simulink model "chap04_CA2"  (R2021a)
settings: Solver=FixedStepDiscrete  StartTime=0.0  StopTime=30  FixedStep=0.001  RelTol=1e-3
undefined symbols (not defined in the file): DiscIntNeverNeededParam
libraries: simulink x4
(part 3 of 3)

== system chap04_CA2/Subsystem/Subsystem5/Subsystem6 ==
  xx3 : Inport
  xx1 : Inport  Port=2
  xx4 : Inport  Port=3
  xx5 : Inport  Port=4
  vx3 : Inport  Port=5
  vx1 : Inport  Port=6
  vx4 : Inport  Port=7
  vx5 : Inport  Port=8
  Add : Sum
  Add{1,4,6,8} (4 alike) : Sum  Inputs=-+
  Add2 : Sum  Inputs=+-
  Add5 : Sum  Inputs=+++
  Add7 : Sum  Inputs=+-
  Add9 : Sum  Inputs=+++
  Constant{,1,3,6} (4 alike) : Constant  Value=1.0
  Constant2 : Constant  Value=7/9
  Constant4 : Constant  Value=0.5
  Constant5 : Constant  Value=1.5
  Constant7 : Constant  Value=0.5
  Constant8 : Constant  Value=1.5
  Constant9 : Constant  Value=3
  Divide : Product  Inputs=*/
  Gain : Gain  Gain=-1
  Math Function1 : Math  Operator=pow  SignedPower=on  SaturateOnIntegerOverflow=on
  Product{1,3..9} (8 alike) : Product
  p3x : Outport
  wires:
  Product8/1 -> Add9/2
  Product9/1 -> Add9/3
  Constant6/1 -> Product8/1
  Add8/1 -> Product8/2
  vx3/1 -> Add6/2, Add8/2, Add7/1
  Constant7/1 -> Product9/2
  Add7/1 -> Product9/1
  vx4/1 -> Add8/1
  vx1/1 -> Add7/2
  vx5/1 -> Add6/1
  Constant8/1 -> Product7/1
  Add6/1 -> Product7/2
  Product7/1 -> Add9/1
  Product3/1 -> Add5/1
  Add1/1 -> Product3/2
  Constant5/1 -> Product3/1
  xx5/1 -> Add1/1
  xx1/1 -> Add2/2
  xx4/1 -> Add4/1
  Add5/1 -> Product6/2
  Add2/1 -> Product5/1
  Product1/1 -> Add/2
  Constant1/1 -> Product1/1
  Constant/1 -> Product6/1
  Product6/1 -> Add/1
  Constant4/1 -> Product5/2
  xx3/1 -> Add2/1, Add4/2, Add1/2
  Add4/1 -> Product4/2
  Constant3/1 -> Product4/1
  Product5/1 -> Add5/3
  Product4/1 -> Add5/2
  Add9/1 -> Product1/2
  Math Function1/1 -> Gain/1
  Constant9/1 -> Divide/2
  Divide/1 -> Math Function1/1
  Add/1 -> Divide/1
  Constant2/1 -> Math Function1/2
  Gain/1 -> p3x/1

== system chap04_CA2/Subsystem/Subsystem5/Subsystem7 ==
  vy3 : Inport
  uty : Inport  Port=2
  gain : Inport  Port=3
  Add1 : Sum  Inputs=--+
  Constant : Constant  Value=0.08
  Constant2 : Constant  Value=15
  Product : Product
  Product1 : Product
  Product2 : Product
  Subsystem : Subsystem
  Subtract : Sum  Inputs=+-
  Tanh : Trigonometry  Operator=tanh
  ux : Outport
  wires:
  Subtract/1 -> Product2/1, Product1/2
  Constant/1 -> Product1/1
  Product1/1 -> Add1/1
  Constant2/1 -> Product2/2
  [A] -> Add1/3
  gain/1 -> Product/2
  Tanh/1 -> Product/1
  Product2/1 -> Tanh/1
  vy3/1 -> Subtract/1
  Product/1 -> Add1/2
  Subsystem/1(Out1) -> Subtract/2
  uty/1 -> Subsystem/1(zt3), [A]
  Add1/1 -> ux/1

== system chap04_CA2/Subsystem/Subsystem5/Subsystem8 ==
  vz3 : Inport
  utz : Inport  Port=2
  gain : Inport  Port=3
  Add1 : Sum  Inputs=--+
  Constant : Constant  Value=0.08
  Constant2 : Constant  Value=15
  Product : Product
  Product1 : Product
  Product2 : Product
  Subsystem : Subsystem
  Subtract : Sum  Inputs=+-
  Tanh : Trigonometry  Operator=tanh
  ux : Outport
  wires:
  Add1/1 -> ux/1
  utz/1 -> [A], Subsystem/1(zt3)
  Subsystem/1(Out1) -> Subtract/2
  Product/1 -> Add1/2
  vz3/1 -> Subtract/1
  Product2/1 -> Tanh/1
  Tanh/1 -> Product/1
  gain/1 -> Product/2
  [A] -> Add1/3
  Constant2/1 -> Product2/2
  Product1/1 -> Add1/1
  Constant/1 -> Product1/1
  Subtract/1 -> Product1/2, Product2/1

== system chap04_CA2/Subsystem2/Subsystem7/Subsystem1 ==
  Abs1 : Abs
  Add : Sum  Inputs=+++
  Constant : Constant  Value=0.8
  Constant1 : Constant  Value=0.1
  Constant3 : Constant  Value=0.1
  Delay1 : Delay
  Delay2 : Delay  DelayLength=1
  Product{1..4} (4 alike) : Product
  Random Number1 : RandomNumber  Mean=0.75  Variance=0.5  Seed=2  SampleTime=0.01
  Repeating Sequence Interpolated2 : simulink/Sources/Repeating Sequence Interpolated  OutValues=[0.5 0.25 0.4 0.35 0.1].'  TimeValues=[0 0.1 0.5 0.6 1].'  LookUpMeth=Use Input Nearest  tsamp=1  OutMin=[]  OutMax=[]  OutDataTypeStr=double  OutputDataTypeScalingMode=double  OutDataType=fixdt(0,8)  OutScaling=2^-10
  Scope : Scope
  Out2 : Outport
  wires:
  Delay1/1 -> Product2/1
  Delay2/1 -> Product1/1
  Constant/1 -> Product2/2
  Constant3/1 -> Product1/2
  Constant1/1 -> Product3/2
  Product3/1 -> Add/1
  Product1/1 -> Add/2
  Product2/1 -> Add/3
  Product4/1 -> Product3/1
  Add/1 -> Out2/1, Delay1/1, Delay2/1
  Abs1/1 -> Product4/1, Scope/1
  Random Number1/1 -> Abs1/1
  Repeating Sequence Interpolated2/1 -> Product4/2

== system chap04_CA2/Subsystem2/Subsystem7/Subsystem2 ==
  In2 : Inport
  Add : Sum  Inputs=+++
  Constant : Constant  Value=0.8
  Constant1 : Constant  Value=0.1
  Constant3 : Constant  Value=0.1
  Delay1 : Delay
  Delay2 : Delay  DelayLength=1
  Product1 : Product
  Product2 : Product
  Product3 : Product
  Out2 : Outport
  wires:
  Add/1 -> Delay2/1, Delay1/1, Out2/1
  In2/1 -> Product3/1
  Product2/1 -> Add/3
  Product1/1 -> Add/2
  Product3/1 -> Add/1
  Constant1/1 -> Product3/2
  Constant3/1 -> Product1/2
  Constant/1 -> Product2/2
  Delay2/1 -> Product1/1
  Delay1/1 -> Product2/1

== system chap04_CA2/Subsystem2/Subsystem7/Subsystem3 ==
  In2 : Inport
  Add : Sum  Inputs=+++
  Constant : Constant  Value=0.8
  Constant1 : Constant  Value=0.1
  Constant3 : Constant  Value=0.1
  Delay1 : Delay
  Delay2 : Delay  DelayLength=1
  Product1 : Product
  Product2 : Product
  Product3 : Product
  Out2 : Outport
  wires:
  Delay1/1 -> Product2/1
  Delay2/1 -> Product1/1
  Constant/1 -> Product2/2
  Constant3/1 -> Product1/2
  Constant1/1 -> Product3/2
  Product3/1 -> Add/1
  Product1/1 -> Add/2
  Product2/1 -> Add/3
  In2/1 -> Product3/1
  Add/1 -> Out2/1, Delay1/1, Delay2/1

== system chap04_CA2/Subsystem2/Subsystem7/Subsystem4 ==
  In2 : Inport
  Add : Sum  Inputs=+++
  Constant : Constant  Value=0.8
  Constant1 : Constant  Value=0.1
  Constant3 : Constant  Value=0.1
  Delay1 : Delay
  Delay2 : Delay  DelayLength=1
  Product1 : Product
  Product2 : Product
  Product3 : Product
  Out2 : Outport
  wires:
  Add/1 -> Delay2/1, Delay1/1, Out2/1
  In2/1 -> Product3/1
  Product2/1 -> Add/3
  Product1/1 -> Add/2
  Product3/1 -> Add/1
  Constant1/1 -> Product3/2
  Constant3/1 -> Product1/2
  Constant/1 -> Product2/2
  Delay2/1 -> Product1/1
  Delay1/1 -> Product2/1

== system chap04_CA2/Subsystem/Subsystem/Subsystem4/Subsystem ==
  zt3 : Inport
  Constant4 : Constant  Value=0
  Discrete-Time Integrator : DiscreteIntegrator  SampleTime=-1  UpperSaturationLimit=100  LowerSaturationLimit=-100  ICPrevOutput=DiscIntNeverNeededParam  ICPrevScaledInput=DiscIntNeverNeededParam
  Logical Operator : Logic  AllPortsSameDT=off  OutDataTypeStr=boolean
  MATLAB Function : MATLAB Function  TreatAsAtomicUnit=on
  Relational Operator : RelationalOperator  Operator===  OutDataTypeStr=boolean  RndMeth=Simplest
  Saturation : Saturate  UpperLimit=5  LowerLimit=-5
  Sign : Signum
  Sign1 : Signum
  Switch : Switch  Criteria=u2 > Threshold
  Out1 : Outport
  wires:
  MATLAB Function/1(y) -> Logical Operator/1
  Relational Operator/1 -> Logical Operator/2
  Constant4/1 -> Switch/1
  Sign1/1 -> Relational Operator/1
  zt3/1 -> Sign1/1, Switch/3
  Saturation/1 -> Out1/1, MATLAB Function/2(u2)
  Discrete-Time Integrator/1 -> Saturation/1, MATLAB Function/1(u1), Sign/1
  Sign/1 -> Relational Operator/2
  Logical Operator/1 -> Switch/2
  Switch/1 -> Discrete-Time Integrator/1

== system chap04_CA2/Subsystem/Subsystem/Subsystem7/Subsystem ==
  zt3 : Inport
  Constant4 : Constant  Value=0
  Discrete-Time Integrator : DiscreteIntegrator  SampleTime=-1  UpperSaturationLimit=100  LowerSaturationLimit=-100  ICPrevOutput=DiscIntNeverNeededParam  ICPrevScaledInput=DiscIntNeverNeededParam
  Logical Operator : Logic  AllPortsSameDT=off  OutDataTypeStr=boolean
  MATLAB Function : MATLAB Function  TreatAsAtomicUnit=on
  Relational Operator : RelationalOperator  Operator===  OutDataTypeStr=boolean  RndMeth=Simplest
  Saturation : Saturate  UpperLimit=5  LowerLimit=-5
  Sign : Signum
  Sign1 : Signum
  Switch : Switch  Criteria=u2 > Threshold
  Out1 : Outport
  wires:
  Switch/1 -> Discrete-Time Integrator/1
  Logical Operator/1 -> Switch/2
  Sign/1 -> Relational Operator/2
  Discrete-Time Integrator/1 -> Sign/1, MATLAB Function/1(u1), Saturation/1
  Saturation/1 -> MATLAB Function/2(u2), Out1/1
  zt3/1 -> Switch/3, Sign1/1
  Sign1/1 -> Relational Operator/1
  Constant4/1 -> Switch/1
  Relational Operator/1 -> Logical Operator/2
  MATLAB Function/1(y) -> Logical Operator/1

== system chap04_CA2/Subsystem/Subsystem/Subsystem8/Subsystem ==
  zt3 : Inport
  Constant4 : Constant  Value=0
  Discrete-Time Integrator : DiscreteIntegrator  SampleTime=-1  UpperSaturationLimit=100  LowerSaturationLimit=-100  ICPrevOutput=DiscIntNeverNeededParam  ICPrevScaledInput=DiscIntNeverNeededParam
  Logical Operator : Logic  AllPortsSameDT=off  OutDataTypeStr=boolean
  MATLAB Function : MATLAB Function  TreatAsAtomicUnit=on
  Relational Operator : RelationalOperator  Operator===  OutDataTypeStr=boolean  RndMeth=Simplest
  Saturation : Saturate  UpperLimit=5  LowerLimit=-5
  Sign : Signum
  Sign1 : Signum
  Switch : Switch  Criteria=u2 > Threshold
  Out1 : Outport
  wires:
  MATLAB Function/1(y) -> Logical Operator/1
  Relational Operator/1 -> Logical Operator/2
  Constant4/1 -> Switch/1
  Sign1/1 -> Relational Operator/1
  zt3/1 -> Sign1/1, Switch/3
  Saturation/1 -> Out1/1, MATLAB Function/2(u2)
  Discrete-Time Integrator/1 -> Saturation/1, MATLAB Function/1(u1), Sign/1
  Sign/1 -> Relational Operator/2
  Logical Operator/1 -> Switch/2
  Switch/1 -> Discrete-Time Integrator/1

== system chap04_CA2/Subsystem/Subsystem1/Subsystem4/Subsystem ==
  zt3 : Inport
  Constant4 : Constant  Value=0
  Discrete-Time Integrator : DiscreteIntegrator  SampleTime=-1  UpperSaturationLimit=100  LowerSaturationLimit=-100  ICPrevOutput=DiscIntNeverNeededParam  ICPrevScaledInput=DiscIntNeverNeededParam
  Logical Operator : Logic  AllPortsSameDT=off  OutDataTypeStr=boolean
  MATLAB Function : MATLAB Function  TreatAsAtomicUnit=on
  Relational Operator : RelationalOperator  Operator===  OutDataTypeStr=boolean  RndMeth=Simplest
  Saturation : Saturate  UpperLimit=5  LowerLimit=-5
  Sign : Signum
  Sign1 : Signum
  Switch : Switch  Criteria=u2 > Threshold
  Out1 : Outport
  wires:
  MATLAB Function/1(y) -> Logical Operator/1
  Relational Operator/1 -> Logical Operator/2
  Constant4/1 -> Switch/1
  Sign1/1 -> Relational Operator/1
  zt3/1 -> Sign1/1, Switch/3
  Saturation/1 -> Out1/1, MATLAB Function/2(u2)
  Discrete-Time Integrator/1 -> Saturation/1, MATLAB Function/1(u1), Sign/1
  Sign/1 -> Relational Operator/2
  Logical Operator/1 -> Switch/2
  Switch/1 -> Discrete-Time Integrator/1

== system chap04_CA2/Subsystem/Subsystem1/Subsystem7/Subsystem ==
  zt3 : Inport
  Constant4 : Constant  Value=0
  Discrete-Time Integrator : DiscreteIntegrator  SampleTime=-1  UpperSaturationLimit=100  LowerSaturationLimit=-100  ICPrevOutput=DiscIntNeverNeededParam  ICPrevScaledInput=DiscIntNeverNeededParam
  Logical Operator : Logic  AllPortsSameDT=off  OutDataTypeStr=boolean
  MATLAB Function : MATLAB Function  TreatAsAtomicUnit=on
  Relational Operator : RelationalOperator  Operator===  OutDataTypeStr=boolean  RndMeth=Simplest
  Saturation : Saturate  UpperLimit=5  LowerLimit=-5
  Sign : Signum
  Sign1 : Signum
  Switch : Switch  Criteria=u2 > Threshold
  Out1 : Outport
  wires:
  Switch/1 -> Discrete-Time Integrator/1
  Logical Operator/1 -> Switch/2
  Sign/1 -> Relational Operator/2
  Discrete-Time Integrator/1 -> Sign/1, MATLAB Function/1(u1), Saturation/1
  Saturation/1 -> MATLAB Function/2(u2), Out1/1
  zt3/1 -> Switch/3, Sign1/1
  Sign1/1 -> Relational Operator/1
  Constant4/1 -> Switch/1
  Relational Operator/1 -> Logical Operator/2
  MATLAB Function/1(y) -> Logical Operator/1

== system chap04_CA2/Subsystem/Subsystem1/Subsystem8/Subsystem ==
  zt3 : Inport
  Constant4 : Constant  Value=0
  Discrete-Time Integrator : DiscreteIntegrator  SampleTime=-1  UpperSaturationLimit=100  LowerSaturationLimit=-100  ICPrevOutput=DiscIntNeverNeededParam  ICPrevScaledInput=DiscIntNeverNeededParam
  Logical Operator : Logic  AllPortsSameDT=off  OutDataTypeStr=boolean
  MATLAB Function : MATLAB Function  TreatAsAtomicUnit=on
  Relational Operator : RelationalOperator  Operator===  OutDataTypeStr=boolean  RndMeth=Simplest
  Saturation : Saturate  UpperLimit=5  LowerLimit=-5
  Sign : Signum
  Sign1 : Signum
  Switch : Switch  Criteria=u2 > Threshold
  Out1 : Outport
  wires:
  MATLAB Function/1(y) -> Logical Operator/1
  Relational Operator/1 -> Logical Operator/2
  Constant4/1 -> Switch/1
  Sign1/1 -> Relational Operator/1
  zt3/1 -> Sign1/1, Switch/3
  Saturation/1 -> Out1/1, MATLAB Function/2(u2)
  Discrete-Time Integrator/1 -> Saturation/1, MATLAB Function/1(u1), Sign/1
  Sign/1 -> Relational Operator/2
  Logical Operator/1 -> Switch/2
  Switch/1 -> Discrete-Time Integrator/1

== system chap04_CA2/Subsystem/Subsystem2/Subsystem4/Subsystem ==
  zt3 : Inport
  Constant4 : Constant  Value=0
  Discrete-Time Integrator : DiscreteIntegrator  SampleTime=-1  UpperSaturationLimit=100  LowerSaturationLimit=-100  ICPrevOutput=DiscIntNeverNeededParam  ICPrevScaledInput=DiscIntNeverNeededParam
  Logical Operator : Logic  AllPortsSameDT=off  OutDataTypeStr=boolean
  MATLAB Function : MATLAB Function  TreatAsAtomicUnit=on
  Relational Operator : RelationalOperator  Operator===  OutDataTypeStr=boolean  RndMeth=Simplest
  Saturation : Saturate  UpperLimit=5  LowerLimit=-5
  Sign : Signum
  Sign1 : Signum
  Switch : Switch  Criteria=u2 > Threshold
  Out1 : Outport
  wires:
  MATLAB Function/1(y) -> Logical Operator/1
  Relational Operator/1 -> Logical Operator/2
  Constant4/1 -> Switch/1
  Sign1/1 -> Relational Operator/1
  zt3/1 -> Sign1/1, Switch/3
  Saturation/1 -> Out1/1, MATLAB Function/2(u2)
  Discrete-Time Integrator/1 -> Saturation/1, MATLAB Function/1(u1), Sign/1
  Sign/1 -> Relational Operator/2
  Logical Operator/1 -> Switch/2
  Switch/1 -> Discrete-Time Integrator/1

== system chap04_CA2/Subsystem/Subsystem2/Subsystem7/Subsystem ==
  zt3 : Inport
  Constant4 : Constant  Value=0
  Discrete-Time Integrator : DiscreteIntegrator  SampleTime=-1  UpperSaturationLimit=100  LowerSaturationLimit=-100  ICPrevOutput=DiscIntNeverNeededParam  ICPrevScaledInput=DiscIntNeverNeededParam
  Logical Operator : Logic  AllPortsSameDT=off  OutDataTypeStr=boolean
  MATLAB Function : MATLAB Function  TreatAsAtomicUnit=on
  Relational Operator : RelationalOperator  Operator===  OutDataTypeStr=boolean  RndMeth=Simplest
  Saturation : Saturate  UpperLimit=5  LowerLimit=-5
  Sign : Signum
  Sign1 : Signum
  Switch : Switch  Criteria=u2 > Threshold
  Out1 : Outport
  wires:
  Switch/1 -> Discrete-Time Integrator/1
  Logical Operator/1 -> Switch/2
  Sign/1 -> Relational Operator/2
  Discrete-Time Integrator/1 -> Sign/1, MATLAB Function/1(u1), Saturation/1
  Saturation/1 -> MATLAB Function/2(u2), Out1/1
  zt3/1 -> Switch/3, Sign1/1
  Sign1/1 -> Relational Operator/1
  Constant4/1 -> Switch/1
  Relational Operator/1 -> Logical Operator/2
  MATLAB Function/1(y) -> Logical Operator/1

== system chap04_CA2/Subsystem/Subsystem2/Subsystem8/Subsystem ==
  zt3 : Inport
  Constant4 : Constant  Value=0
  Discrete-Time Integrator : DiscreteIntegrator  SampleTime=-1  UpperSaturationLimit=100  LowerSaturationLimit=-100  ICPrevOutput=DiscIntNeverNeededParam  ICPrevScaledInput=DiscIntNeverNeededParam
  Logical Operator : Logic  AllPortsSameDT=off  OutDataTypeStr=boolean
  MATLAB Function : MATLAB Function  TreatAsAtomicUnit=on
  Relational Operator : RelationalOperator  Operator===  OutDataTypeStr=boolean  RndMeth=Simplest
  Saturation : Saturate  UpperLimit=5  LowerLimit=-5
  Sign : Signum
  Sign1 : Signum
  Switch : Switch  Criteria=u2 > Threshold
  Out1 : Outport
  wires:
  MATLAB Function/1(y) -> Logical Operator/1
  Relational Operator/1 -> Logical Operator/2
  Constant4/1 -> Switch/1
  Sign1/1 -> Relational Operator/1
  zt3/1 -> Sign1/1, Switch/3
  Saturation/1 -> Out1/1, MATLAB Function/2(u2)
  Discrete-Time Integrator/1 -> Saturation/1, MATLAB Function/1(u1), Sign/1
  Sign/1 -> Relational Operator/2
  Logical Operator/1 -> Switch/2
  Switch/1 -> Discrete-Time Integrator/1

== system chap04_CA2/Subsystem/Subsystem3/Subsystem4/Subsystem ==
  zt3 : Inport
  Constant4 : Constant  Value=0
  Discrete-Time Integrator : DiscreteIntegrator  SampleTime=-1  UpperSaturationLimit=100  LowerSaturationLimit=-100  ICPrevOutput=DiscIntNeverNeededParam  ICPrevScaledInput=DiscIntNeverNeededParam
  Logical Operator : Logic  AllPortsSameDT=off  OutDataTypeStr=boolean
  MATLAB Function : MATLAB Function  TreatAsAtomicUnit=on
  Relational Operator : RelationalOperator  Operator===  OutDataTypeStr=boolean  RndMeth=Simplest
  Saturation : Saturate  UpperLimit=5  LowerLimit=-5
  Sign : Signum
  Sign1 : Signum
  Switch : Switch  Criteria=u2 > Threshold
  Out1 : Outport
  wires:
  MATLAB Function/1(y) -> Logical Operator/1
  Relational Operator/1 -> Logical Operator/2
  Constant4/1 -> Switch/1
  Sign1/1 -> Relational Operator/1
  zt3/1 -> Sign1/1, Switch/3
  Saturation/1 -> Out1/1, MATLAB Function/2(u2)
  Discrete-Time Integrator/1 -> Saturation/1, MATLAB Function/1(u1), Sign/1
  Sign/1 -> Relational Operator/2
  Logical Operator/1 -> Switch/2
  Switch/1 -> Discrete-Time Integrator/1

== system chap04_CA2/Subsystem/Subsystem3/Subsystem7/Subsystem ==
  zt3 : Inport
  Constant4 : Constant  Value=0
  Discrete-Time Integrator : DiscreteIntegrator  SampleTime=-1  UpperSaturationLimit=100  LowerSaturationLimit=-100  ICPrevOutput=DiscIntNeverNeededParam  ICPrevScaledInput=DiscIntNeverNeededParam
  Logical Operator : Logic  AllPortsSameDT=off  OutDataTypeStr=boolean
  MATLAB Function : MATLAB Function  TreatAsAtomicUnit=on
  Relational Operator : RelationalOperator  Operator===  OutDataTypeStr=boolean  RndMeth=Simplest
  Saturation : Saturate  UpperLimit=5  LowerLimit=-5
  Sign : Signum
  Sign1 : Signum
  Switch : Switch  Criteria=u2 > Threshold
  Out1 : Outport
  wires:
  Switch/1 -> Discrete-Time Integrator/1
  Logical Operator/1 -> Switch/2
  Sign/1 -> Relational Operator/2
  Discrete-Time Integrator/1 -> Sign/1, MATLAB Function/1(u1), Saturation/1
  Saturation/1 -> MATLAB Function/2(u2), Out1/1
  zt3/1 -> Switch/3, Sign1/1
  Sign1/1 -> Relational Operator/1
  Constant4/1 -> Switch/1
  Relational Operator/1 -> Logical Operator/2
  MATLAB Function/1(y) -> Logical Operator/1

== system chap04_CA2/Subsystem/Subsystem3/Subsystem8/Subsystem ==
  zt3 : Inport
  Constant4 : Constant  Value=0
  Discrete-Time Integrator : DiscreteIntegrator  SampleTime=-1  UpperSaturationLimit=100  LowerSaturationLimit=-100  ICPrevOutput=DiscIntNeverNeededParam  ICPrevScaledInput=DiscIntNeverNeededParam
  Logical Operator : Logic  AllPortsSameDT=off  OutDataTypeStr=boolean
  MATLAB Function : MATLAB Function  TreatAsAtomicUnit=on
  Relational Operator : RelationalOperator  Operator===  OutDataTypeStr=boolean  RndMeth=Simplest
  Saturation : Saturate  UpperLimit=5  LowerLimit=-5
  Sign : Signum
  Sign1 : Signum
  Switch : Switch  Criteria=u2 > Threshold
  Out1 : Outport
  wires:
  MATLAB Function/1(y) -> Logical Operator/1
  Relational Operator/1 -> Logical Operator/2
  Constant4/1 -> Switch/1
  Sign1/1 -> Relational Operator/1
  zt3/1 -> Sign1/1, Switch/3
  Saturation/1 -> Out1/1, MATLAB Function/2(u2)
  Discrete-Time Integrator/1 -> Saturation/1, MATLAB Function/1(u1), Sign/1
  Sign/1 -> Relational Operator/2
  Logical Operator/1 -> Switch/2
  Switch/1 -> Discrete-Time Integrator/1

== system chap04_CA2/Subsystem/Subsystem4/Subsystem4/Subsystem ==
  zt3 : Inport
  Constant4 : Constant  Value=0
  Discrete-Time Integrator : DiscreteIntegrator  SampleTime=-1  UpperSaturationLimit=100  LowerSaturationLimit=-100  ICPrevOutput=DiscIntNeverNeededParam  ICPrevScaledInput=DiscIntNeverNeededParam
  Logical Operator : Logic  AllPortsSameDT=off  OutDataTypeStr=boolean
  MATLAB Function : MATLAB Function  TreatAsAtomicUnit=on
  Relational Operator : RelationalOperator  Operator===  OutDataTypeStr=boolean  RndMeth=Simplest
  Saturation : Saturate  UpperLimit=5  LowerLimit=-5
  Sign : Signum
  Sign1 : Signum
  Switch : Switch  Criteria=u2 > Threshold
  Out1 : Outport
  wires:
  MATLAB Function/1(y) -> Logical Operator/1
  Relational Operator/1 -> Logical Operator/2
  Constant4/1 -> Switch/1
  Sign1/1 -> Relational Operator/1
  zt3/1 -> Sign1/1, Switch/3
  Saturation/1 -> Out1/1, MATLAB Function/2(u2)
  Discrete-Time Integrator/1 -> Saturation/1, MATLAB Function/1(u1), Sign/1
  Sign/1 -> Relational Operator/2
  Logical Operator/1 -> Switch/2
  Switch/1 -> Discrete-Time Integrator/1

== system chap04_CA2/Subsystem/Subsystem4/Subsystem7/Subsystem ==
  zt3 : Inport
  Constant4 : Constant  Value=0
  Discrete-Time Integrator : DiscreteIntegrator  SampleTime=-1  UpperSaturationLimit=100  LowerSaturationLimit=-100  ICPrevOutput=DiscIntNeverNeededParam  ICPrevScaledInput=DiscIntNeverNeededParam
  Logical Operator : Logic  AllPortsSameDT=off  OutDataTypeStr=boolean
  MATLAB Function : MATLAB Function  TreatAsAtomicUnit=on
  Relational Operator : RelationalOperator  Operator===  OutDataTypeStr=boolean  RndMeth=Simplest
  Saturation : Saturate  UpperLimit=5  LowerLimit=-5
  Sign : Signum
  Sign1 : Signum
  Switch : Switch  Criteria=u2 > Threshold
  Out1 : Outport
  wires:
  Switch/1 -> Discrete-Time Integrator/1
  Logical Operator/1 -> Switch/2
  Sign/1 -> Relational Operator/2
  Discrete-Time Integrator/1 -> Sign/1, MATLAB Function/1(u1), Saturation/1
  Saturation/1 -> MATLAB Function/2(u2), Out1/1
  zt3/1 -> Switch/3, Sign1/1
  Sign1/1 -> Relational Operator/1
  Constant4/1 -> Switch/1
  Relational Operator/1 -> Logical Operator/2
  MATLAB Function/1(y) -> Logical Operator/1

== system chap04_CA2/Subsystem/Subsystem4/Subsystem8/Subsystem ==
  zt3 : Inport
  Constant4 : Constant  Value=0
  Discrete-Time Integrator : DiscreteIntegrator  SampleTime=-1  UpperSaturationLimit=100  LowerSaturationLimit=-100  ICPrevOutput=DiscIntNeverNeededParam  ICPrevScaledInput=DiscIntNeverNeededParam
  Logical Operator : Logic  AllPortsSameDT=off  OutDataTypeStr=boolean
  MATLAB Function : MATLAB Function  TreatAsAtomicUnit=on
  Relational Operator : RelationalOperator  Operator===  OutDataTypeStr=boolean  RndMeth=Simplest
  Saturation : Saturate  UpperLimit=5  LowerLimit=-5
  Sign : Signum
  Sign1 : Signum
  Switch : Switch  Criteria=u2 > Threshold
  Out1 : Outport
  wires:
  MATLAB Function/1(y) -> Logical Operator/1
  Relational Operator/1 -> Logical Operator/2
  Constant4/1 -> Switch/1
  Sign1/1 -> Relational Operator/1
  zt3/1 -> Sign1/1, Switch/3
  Saturation/1 -> Out1/1, MATLAB Function/2(u2)
  Discrete-Time Integrator/1 -> Saturation/1, MATLAB Function/1(u1), Sign/1
  Sign/1 -> Relational Operator/2
  Logical Operator/1 -> Switch/2
  Switch/1 -> Discrete-Time Integrator/1

== system chap04_CA2/Subsystem/Subsystem5/Subsystem4/Subsystem ==
  zt3 : Inport
  Constant4 : Constant  Value=0
  Discrete-Time Integrator : DiscreteIntegrator  SampleTime=-1  UpperSaturationLimit=100  LowerSaturationLimit=-100  ICPrevOutput=DiscIntNeverNeededParam  ICPrevScaledInput=DiscIntNeverNeededParam
  Logical Operator : Logic  AllPortsSameDT=off  OutDataTypeStr=boolean
  MATLAB Function : MATLAB Function  TreatAsAtomicUnit=on
  Relational Operator : RelationalOperator  Operator===  OutDataTypeStr=boolean  RndMeth=Simplest
  Saturation : Saturate  UpperLimit=5  LowerLimit=-5
  Sign : Signum
  Sign1 : Signum
  Switch : Switch  Criteria=u2 > Threshold
  Out1 : Outport
  wires:
  MATLAB Function/1(y) -> Logical Operator/1
  Relational Operator/1 -> Logical Operator/2
  Constant4/1 -> Switch/1
  Sign1/1 -> Relational Operator/1
  zt3/1 -> Sign1/1, Switch/3
  Saturation/1 -> Out1/1, MATLAB Function/2(u2)
  Discrete-Time Integrator/1 -> Saturation/1, MATLAB Function/1(u1), Sign/1
  Sign/1 -> Relational Operator/2
  Logical Operator/1 -> Switch/2
  Switch/1 -> Discrete-Time Integrator/1

== system chap04_CA2/Subsystem/Subsystem5/Subsystem7/Subsystem ==
  zt3 : Inport
  Constant4 : Constant  Value=0
  Discrete-Time Integrator : DiscreteIntegrator  SampleTime=-1  UpperSaturationLimit=100  LowerSaturationLimit=-100  ICPrevOutput=DiscIntNeverNeededParam  ICPrevScaledInput=DiscIntNeverNeededParam
  Logical Operator : Logic  AllPortsSameDT=off  OutDataTypeStr=boolean
  MATLAB Function : MATLAB Function  TreatAsAtomicUnit=on
  Relational Operator : RelationalOperator  Operator===  OutDataTypeStr=boolean  RndMeth=Simplest
  Saturation : Saturate  UpperLimit=5  LowerLimit=-5
  Sign : Signum
  Sign1 : Signum
  Switch : Switch  Criteria=u2 > Threshold
  Out1 : Outport
  wires:
  Switch/1 -> Discrete-Time Integrator/1
  Logical Operator/1 -> Switch/2
  Sign/1 -> Relational Operator/2
  Discrete-Time Integrator/1 -> Sign/1, MATLAB Function/1(u1), Saturation/1
  Saturation/1 -> MATLAB Function/2(u2), Out1/1
  zt3/1 -> Switch/3, Sign1/1
  Sign1/1 -> Relational Operator/1
  Constant4/1 -> Switch/1
  Relational Operator/1 -> Logical Operator/2
  MATLAB Function/1(y) -> Logical Operator/1

== system chap04_CA2/Subsystem/Subsystem5/Subsystem8/Subsystem ==
  zt3 : Inport
  Constant4 : Constant  Value=0
  Discrete-Time Integrator : DiscreteIntegrator  SampleTime=-1  UpperSaturationLimit=100  LowerSaturationLimit=-100  ICPrevOutput=DiscIntNeverNeededParam  ICPrevScaledInput=DiscIntNeverNeededParam
  Logical Operator : Logic  AllPortsSameDT=off  OutDataTypeStr=boolean
  MATLAB Function : MATLAB Function  TreatAsAtomicUnit=on
  Relational Operator : RelationalOperator  Operator===  OutDataTypeStr=boolean  RndMeth=Simplest
  Saturation : Saturate  UpperLimit=5  LowerLimit=-5
  Sign : Signum
  Sign1 : Signum
  Switch : Switch  Criteria=u2 > Threshold
  Out1 : Outport
  wires:
  MATLAB Function/1(y) -> Logical Operator/1
  Relational Operator/1 -> Logical Operator/2
  Constant4/1 -> Switch/1
  Sign1/1 -> Relational Operator/1
  zt3/1 -> Sign1/1, Switch/3
  Saturation/1 -> Out1/1, MATLAB Function/2(u2)
  Discrete-Time Integrator/1 -> Saturation/1, MATLAB Function/1(u1), Sign/1
  Sign/1 -> Relational Operator/2
  Logical Operator/1 -> Switch/2
  Switch/1 -> Discrete-Time Integrator/1

== matlab function chap04_CA2/Subsystem/Subsystem5/Subsystem8/Subsystem/MATLAB Function ==
  data: u1 input; y output; u2 input
function y = fcn(u1,u2)


if (u1==u2)
    y = 0;
else
    y = 1;
end

== matlab function chap04_CA2/Subsystem/Subsystem3/Subsystem4/Subsystem/MATLAB Function ==
  data: u1 input; y output; u2 input
function y = fcn(u1,u2)


if (u1==u2)
    y = 0;
else
    y = 1;
end

== matlab function chap04_CA2/Subsystem/Subsystem3/Subsystem7/Subsystem/MATLAB Function ==
  data: u1 input; y output; u2 input
function y = fcn(u1,u2)


if (u1==u2)
    y = 0;
else
    y = 1;
end

== matlab function chap04_CA2/Subsystem/Subsystem4/Subsystem4/Subsystem/MATLAB Function ==
  data: u1 input; y output; u2 input
function y = fcn(u1,u2)


if (u1==u2)
    y = 0;
else
    y = 1;
end

== matlab function chap04_CA2/Subsystem/Subsystem4/Subsystem7/Subsystem/MATLAB Function ==
  data: u1 input; y output; u2 input
function y = fcn(u1,u2)


if (u1==u2)
    y = 0;
else
    y = 1;
end

== matlab function chap04_CA2/Subsystem/Subsystem2/Subsystem4/Subsystem/MATLAB Function ==
  data: u1 input; y output; u2 input
function y = fcn(u1,u2)


if (u1==u2)
    y = 0;
else
    y = 1;
end

== matlab function chap04_CA2/Subsystem/Subsystem4/Subsystem8/Subsystem/MATLAB Function ==
  data: u1 input; y output; u2 input
function y = fcn(u1,u2)


if (u1==u2)
    y = 0;
else
    y = 1;
end

== matlab function chap04_CA2/Subsystem/Subsystem3/Subsystem8/Subsystem/MATLAB Function ==
  data: u1 input; y output; u2 input
function y = fcn(u1,u2)


if (u1==u2)
    y = 0;
else
    y = 1;
end

== matlab function chap04_CA2/Subsystem/Subsystem/Subsystem10/MATLAB Function ==
  data: u input; utk input; nrom output
function nrom = fcn(u,utk)

e = utk-u;
nrom = norm(e);

== matlab function chap04_CA2/Subsystem/Subsystem2/Subsystem10/MATLAB Function ==
  data: u input; utk input; nrom output
function nrom = fcn(u,utk)

e = utk-u;
nrom = norm(e);

== matlab function chap04_CA2/Subsystem/Subsystem5/Subsystem10/MATLAB Function ==
  data: u input; utk input; nrom output
function nrom = fcn(u,utk)

e = utk-u;
nrom = norm(e);

== matlab function chap04_CA2/Subsystem/Subsystem3/Subsystem10/MATLAB Function ==
  data: u input; utk input; nrom output
function nrom = fcn(u,utk)

e = utk-u;
nrom = norm(e);

== matlab function chap04_CA2/Subsystem/Subsystem1/Subsystem10/MATLAB Function ==
  data: u input; utk input; nrom output
function nrom = fcn(u,utk)

e = utk-u;
nrom = norm(e);

== matlab function chap04_CA2/Subsystem/Subsystem4/Subsystem10/MATLAB Function ==
  data: u input; utk input; nrom output
function nrom = fcn(u,utk)

e = utk-u;
nrom = norm(e);

== matlab function chap04_CA2/Subsystem/Subsystem2/Subsystem7/Subsystem/MATLAB Function ==
  data: u1 input; y output; u2 input
function y = fcn(u1,u2)


if (u1==u2)
    y = 0;
else
    y = 1;
end

== matlab function chap04_CA2/Subsystem/Subsystem2/Subsystem8/Subsystem/MATLAB Function ==
  data: u1 input; y output; u2 input
function y = fcn(u1,u2)


if (u1==u2)
    y = 0;
else
    y = 1;
end

== matlab function chap04_CA2/Subsystem/Subsystem1/Subsystem4/Subsystem/MATLAB Function ==
  data: u1 input; y output; u2 input
function y = fcn(u1,u2)


if (u1==u2)
    y = 0;
else
    y = 1;
end

== matlab function chap04_CA2/Subsystem/Subsystem1/Subsystem7/Subsystem/MATLAB Function ==
  data: u1 input; y output; u2 input
function y = fcn(u1,u2)


if (u1==u2)
    y = 0;
else
    y = 1;
end

== matlab function chap04_CA2/Subsystem/Subsystem1/Subsystem8/Subsystem/MATLAB Function ==
  data: u1 input; y output; u2 input
function y = fcn(u1,u2)


if (u1==u2)
    y = 0;
else
    y = 1;
end

== matlab function chap04_CA2/Subsystem/Subsystem/Subsystem7/Subsystem/MATLAB Function ==
  data: u1 input; y output; u2 input
function y = fcn(u1,u2)


if (u1==u2)
    y = 0;
else
    y = 1;
end

== matlab function chap04_CA2/Subsystem/Subsystem/Subsystem8/Subsystem/MATLAB Function ==
  data: u1 input; y output; u2 input
function y = fcn(u1,u2)


if (u1==u2)
    y = 0;
else
    y = 1;
end

== matlab function chap04_CA2/Subsystem/Subsystem/Subsystem4/Subsystem/MATLAB Function ==
  data: u1 input; y output; u2 input
function y = fcn(u1,u2)


if (u1==u2)
    y = 0;
else
    y = 1;
end

== matlab function chap04_CA2/Subsystem/Subsystem5/Subsystem4/Subsystem/MATLAB Function ==
  data: u1 input; y output; u2 input
function y = fcn(u1,u2)


if (u1==u2)
    y = 0;
else
    y = 1;
end

== matlab function chap04_CA2/Subsystem/Subsystem5/Subsystem7/Subsystem/MATLAB Function ==
  data: u1 input; y output; u2 input
function y = fcn(u1,u2)


if (u1==u2)
    y = 0;
else
    y = 1;
end
